simulink model "controlModel"  (R2019b)
settings: Solver=ode3  StartTime=0.0  StopTime=inf  FixedStep=0.01  RelTol=1e-3
PreLoadFcn:
  | controlParams;
values from neighbouring files (symbols this model uses):
  deltaDriftClosed = Simulink.Parameter    [controlParams.m]
  deltaFrac = Simulink.Parameter    [controlParams.m]
  dialVolts = Simulink.Parameter    [controlParams.m]
  IEratioSetting = Simulink.Parameter    [controlParams.m]
  inhaleValveMax = Simulink.Parameter    [controlParams.m]
  modeBPs = Simulink.Parameter    [controlParams.m]
  pressureDynamicRangeSetting = Simulink.Parameter    [controlParams.m]
  pressureEng = Simulink.Parameter    [controlParams.m]
  pressureThresholdMinSetting = Simulink.Parameter    [controlParams.m]
  pressureVolts = Simulink.Parameter    [controlParams.m]
  respRateSetting = Simulink.Parameter    [controlParams.m]
libraries: controlLibrary x4
settings Model: Creator=mwalker  LastModifiedBy=abennett
settings DataIOCC: LimitDataPoints=on  ReturnWorkspaceOutputs=off
settings OptimizationCC: ExpressionDepthLimit=2147483647  LifeSpan=Inf  MaxStackSize=64
settings DebuggingCC: MergeDetectMultiDrivingBlocksExec=none  FcnCallInpInsideContextMsg=warning  AllowSymbolicDim=off  StateNameClashWarn=warning  SFUnexpectedBacktrackingDiag=warning  SFNoUnconditionalDefaultTransitionDiag=warning  SFExecutionAtInitializationDiag=none  ArithmeticOperatorsInVariantConditions=warning
settings HardwareCC: ProdBitPerInt=16  ProdBitPerPointer=16  ProdBitPerSizeT=16  ProdBitPerPtrDiffT=16  ProdLargestAtomicFloat=None  ProdWordSize=8  ProdHWDeviceType=Atmel->AVR  UseEmbeddedCoderFeatures=off  UseSimulinkCoderFeatures=off
settings ModelReferenceCC: PropagateSignalLabelsOutOfModel=off
settings SFSimCC: SimUseLocalCustomCode=off  MATLABDynamicMemAlloc=off
settings RTWCC: SystemTargetFile=ert.tlc  HardwareBoard=Arduino Mega 2560  TemplateMakefile=ert_default_tmf  GenerateReport=on  RTWVerbose=off  RTWUseLocalCustomCode=off  Toolchain=Arduino AVR  BuildConfiguration=Faster Runs  LaunchReport=on
settings CodeAppCC: ForceParamTrailComments=on  OperatorAnnotations=on  StateflowObjectComments=on  MATLABSourceComments=on
settings ERTTargetCC: MultiwordLength=2048  ERTCustomFileBanners=off  SupportContinuousTime=on  SupportNonInlinedSFcns=on  RemoveResetFunc=off  ModelStepFunctionPrototypeControlCompliant=off
settings ConfigComp: CovMetricSettings=dw  CovHtmlReporting=on  CovSaveCumulativeToWorkspaceVar=on  CovSaveSingleToWorkspaceVar=on  CovExternalEMLEnable=off  CovSFcnEnable=off

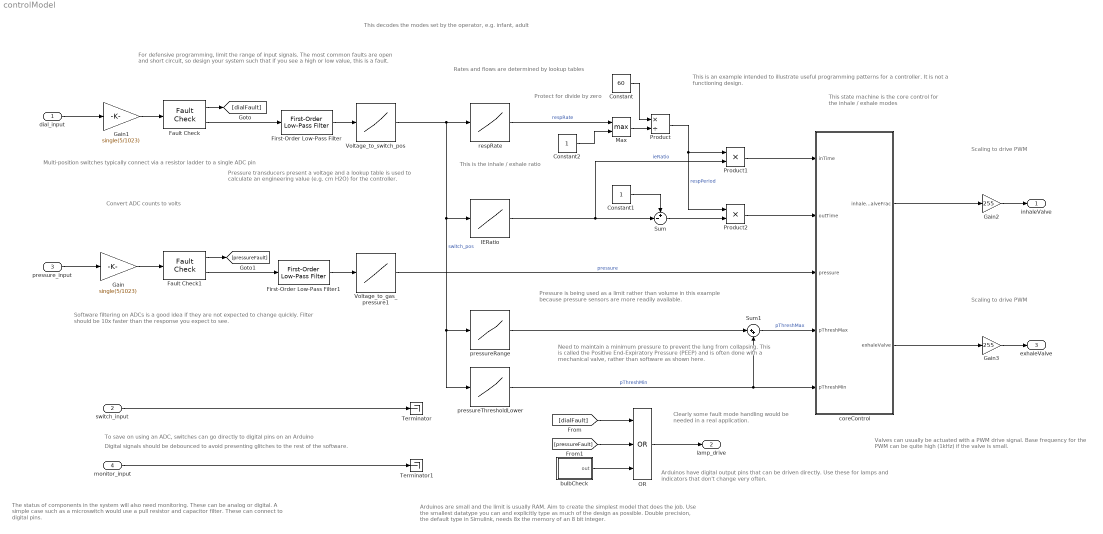
== system controlModel ==
  note: Scaling to drive
      | PWM
  note: Need to maintain a minimum pressure to prevent the lung from collapsing.
      | This is called the Positive End-Expiratory Pressure (PEEP) and is often
      | done with a mechanical valve, rather than software as shown here.
  note: This is an example intended to illustrate useful programming patterns for a controller.
      | It is not a functioning design.
  note: Pressure is being used as a limit rather than volume
      | in this example because pressure sensors are more readily available.
  note: This is the inhale / exhale ratio
  note: This state machine is the core control
      | for the inhale / exhale modes
  note: Clearly some fault mode handling would be
      | needed in a real application.
  note: Protect for divide by zero
  note: Convert ADC counts to volts
  note: Rates and flows are determined by lookup tables
  note: This decodes the modes set by the operator, e.g. infant, adult
  note: For defensive programming, limit the range of input signals. The most common faults are
      | open and short circuit, so design your system such that if you see a high or low value, this
      | is a fault.
  note: Digital signals should be debounced to avoid presenting glitches to the rest of the software.
  note: Software filtering on ADCs is a good idea if they are not expected to change quickly.
      | Filter should be 10x faster than the response you expect to see.
  note: Arduinos are small and the limit is usually RAM. Aim to create the simplest model that does the job.
      | Use the smallest datatype you can and explicitly type as much of the design as possible.
      |
      | Double precision, the default type in Simulink, needs 8x the memory of an 8 bit integer.
  note: Arduinos have digital output pins that can be driven directly. Use these for lamps
      | and indicators that don't change very often.
  note: Valves can usually be actuated with a PWM drive signal.
      | Base frequency for the PWM can be quite high (1kHz) if the valve is small.
  note: The status of components in the system will also need monitoring. These can be analog or digital.
      | A simple case such as a microswitch would use a pull resistor and capacitor filter. These can connect
      | to digital pins.
  note: Pressure transducers present a voltage and a lookup table is used to
      | calculate an engineering value (e.g. cm H2O) for the controller.
  note: To save on using an ADC, switches can go directly to digital pins on an Arduino
  note: Multi-position switches typically connect via a resistor ladder to a single ADC pin
  note: Scaling to drive
      | PWM
  dial_input : Inport  OutDataTypeStr=uint16
  switch_input : Inport  Port=2  OutDataTypeStr=boolean
  pressure_input : Inport  Port=3  OutDataTypeStr=uint16
  monitor_input : Inport  Port=4  OutDataTypeStr=boolean
  Constant : Constant  Value=60  OutDataTypeStr=single
  Constant1 : Constant  OutDataTypeStr=single
  Constant2 : Constant  OutDataTypeStr=single
  Fault Check : controlLibrary/Fault Check  SystemSampleTime=-1  Latency=0  AutoFrameSizeCalculation=off
  Fault Check1 : controlLibrary/Fault Check  SystemSampleTime=-1  Latency=0  AutoFrameSizeCalculation=off
  First-Order Low-Pass Filter : controlLibrary/First-Order Low-Pass Filter  fc=single(0.2)
  First-Order Low-Pass Filter1 : controlLibrary/First-Order Low-Pass Filter  fc=single(0.5)
  Gain : Gain  Gain=single(5/1023)  ParamDataTypeStr=single  OutDataTypeStr=single
  Gain1 : Gain  Gain=single(5/1023)  ParamDataTypeStr=single  OutDataTypeStr=single
  Gain2 : Gain  Gain=255  OutDataTypeStr=uint8
  Gain3 : Gain  Gain=255  OutDataTypeStr=uint8
  IERatio : Lookup_n-D  NumberOfTableDimensions=1  BreakpointsForDimension1=modeBPs  BreakpointsForDimension1DataTypeStr=uint8  Table=IEratioSetting  TableDataTypeStr=single  InterpMethod=Flat  ExtrapMethod=Clip  InternalRulePriority=Speed  OutDataTypeStr=single  RndMeth=Simplest  InputSameDT=on
  Max : MinMax  Function=max  Inputs=2
  OR : Logic  Operator=OR  Inputs=3  AllPortsSameDT=off  OutDataTypeStr=boolean
  Product : Product  Inputs=*/
  Product1 : Product
  Product2 : Product
  Sum : Sum  Inputs=+-|
  Sum1 : Sum  Inputs=|++
  Terminator : Terminator
  Terminator1 : Terminator
  Voltage_to_gas_pressure1 : Lookup_n-D  NumberOfTableDimensions=1  BreakpointsForDimension1=pressureVolts  Table=pressureEng  ExtrapMethod=Clip  InternalRulePriority=Speed  RndMeth=Simplest  InputSameDT=on
  Voltage_to_switch_pos : Lookup_n-D  NumberOfTableDimensions=1  BreakpointsForDimension1=dialVolts  BreakpointsForDimension1DataTypeStr=single  Table=modeBPs  TableDataTypeStr=uint8  InterpMethod=Flat  ExtrapMethod=Clip  InternalRulePriority=Speed  OutDataTypeStr=uint8  RndMeth=Simplest  InputSameDT=on
  bulbCheck : Stateflow chart  BlockKeywords=__PRM__SERIALIZED__DATA__:Stateflow Chart,Stateflow Diagram  TreatAsAtomicUnit=on
  coreControl : Stateflow chart  BlockKeywords=__PRM__SERIALIZED__DATA__:Stateflow Chart,Stateflow Diagram  TreatAsAtomicUnit=on
  pressureRange : Lookup_n-D  NumberOfTableDimensions=1  BreakpointsForDimension1=modeBPs  BreakpointsForDimension1DataTypeStr=uint8  Table=pressureDynamicRangeSetting  TableDataTypeStr=single  InterpMethod=Flat  ExtrapMethod=Clip  InternalRulePriority=Speed  OutDataTypeStr=single  RndMeth=Simplest  InputSameDT=on
  pressureThresholdLower : Lookup_n-D  NumberOfTableDimensions=1  BreakpointsForDimension1=modeBPs  BreakpointsForDimension1DataTypeStr=uint8  Table=pressureThresholdMinSetting  TableDataTypeStr=single  InterpMethod=Flat  ExtrapMethod=Clip  InternalRulePriority=Speed  OutDataTypeStr=single  RndMeth=Simplest  InputSameDT=on
  respRate : Lookup_n-D  NumberOfTableDimensions=1  BreakpointsForDimension1=modeBPs  BreakpointsForDimension1DataTypeStr=uint8  Table=respRateSetting  TableDataTypeStr=single  InterpMethod=Flat  ExtrapMethod=Clip  InternalRulePriority=Speed  OutDataTypeStr=single  RndMeth=Simplest  InputSameDT=on
  inhaleValve : Outport
  lamp_drive : Outport  Port=2
  exhaleValve : Outport  Port=3
  wires:
  pressure_input/1 -> Gain/1
  Fault Check1/2 -> First-Order Low-Pass Filter1/1
  First-Order Low-Pass Filter1/1 -> Voltage_to_gas_pressure1/1
  Voltage_to_gas_pressure1/1 -> coreControl/3(pressure)  "pressure"
  switch_input/1 -> Terminator/1
  dial_input/1 -> Gain1/1
  Fault Check/2 -> First-Order Low-Pass Filter/1
  First-Order Low-Pass Filter/1 -> Voltage_to_switch_pos/1
  Voltage_to_switch_pos/1 -> pressureThresholdLower/1, pressureRange/1, IERatio/1, respRate/1  "switch_pos"
  Fault Check/1 -> [dialFault]
  Fault Check1/1 -> [pressureFault]
  [dialFault] -> OR/1
  [pressureFault] -> OR/2
  OR/1 -> lamp_drive/1
  bulbCheck/1(out) -> OR/3
  respRate/1 -> Max/1  "respRate"
  IERatio/1 -> Sum/2, Product1/2  "ieRatio"
  monitor_input/1 -> Terminator1/1
  Constant/1 -> Product/1
  Product/1 -> Product2/1, Product1/1  "respPeriod"
  Product1/1 -> coreControl/1(inTime)
  Product2/1 -> coreControl/2(outTime)
  Sum/1 -> Product2/2
  Constant1/1 -> Sum/1
  Gain/1 -> Fault Check1/1
  Gain1/1 -> Fault Check/1
  Max/1 -> Product/2
  Constant2/1 -> Max/2
  pressureThresholdLower/1 -> coreControl/5(pThreshMin), Sum1/2  "pThreshMin"
  coreControl/2(exhaleValve) -> Gain3/1
  coreControl/1(inhaleValveFrac) -> Gain2/1
  Gain2/1 -> inhaleValve/1
  Gain3/1 -> exhaleValve/1
  pressureRange/1 -> Sum1/1
  Sum1/1 -> coreControl/4(pThreshMax)  "pThreshMax"

== stateflow chart controlModel/bulbCheck ==
  state BulbCheck
    en: out = true;
  state Run
    en: out = false;
  (default) -> BulbCheck
  BulbCheck -> Run : [after(3,sec)]
  data: out output

== stateflow chart controlModel/coreControl ==
  state Init
    en: exhaleValve = 0;
    inhaleValveFrac=inhaleValveMax;
    inhaleValveMin=0.0;
  note: Initialise inputs and allow to settle
  state IN
    en: inhaleValveFrac = inhaleValveMax;
    exhaleValve = 0;
    count = inTime;
    state PUMP
    state ADJUST
      en: inhaleValveFrac=max(0.0,inhaleValveFrac-deltaFrac);
    (default) -> PUMP
    ADJUST -> PUMP
    PUMP -> ADJUST : [(pressure > pThreshMax) && (inhaleValveFrac>inhaleValveMin)]
  state OUT
    state VENT
      en: count = outTime;
      inhaleValveFrac = 0;
      inhaleValveMin=max(0.0,inhaleValveMin-deltaDriftClosed);
      exhaleValve = 1;
    note: Must also maintain a minimum pressure
    state MAINTAIN_PEEP
      en: exhaleValve = 0;
      inhaleValveMin=inhaleValveMin+deltaFrac;
    (default) -> VENT
    VENT -> MAINTAIN_PEEP : [pressure < pThreshMin]
  (default) -> Init
  Init -> IN : [after(1,sec)]
  OUT -> IN : [after(count,sec)]
  IN -> OUT : [after(count,sec)]
  data: inTime input; count local; outTime input; pressure input; inhaleValveFrac output; pThreshMax input; pThreshMin input; exhaleValve output; inhaleValveMin local; deltaFrac parameter; deltaDriftClosed parameter; inhaleValveMax parameter
